simulink model "gm_uz_pmsm_model_6LUT_pd_vnl"  (R2023a)
settings: Solver=FixedStepAuto  StartTime=0.0  StopTime=0.05  RelTol=1e-3
PreLoadFcn:
  | uz_pmsm_model_init_parameter
PostLoadFcn:
  | % Import the data from Excel for a lookup table
  | FluxMapData = readtable('C:\Users\Philipp\ultrazohm\ultrazohm_sw\ip_cores\uz_pmsm_model\FluxMapData_2023-05-26_13-07-57.csv');
  | % Row indices for lookup table
  | d_current_in_d_axis = FluxMapData(8:27,1:end);
  | % Column indices for lookup table
  | q_current_in_d_axis = FluxMapData(29:48,1:end);
  | % Output values for lookup table
  | d_Flux_d_axis = FluxMapData(50:69,1:end);
undefined symbols (not defined in the file or in its folder): d_current_d_Flux, d_current_q_Flux, entkopplung_dynamic, entkopplung_linear, entkopplung_static, Flux_d, Flux_q, friction_coefficient, inertia, k_i_d, k_p_d, k_p_q, Ki_Bo_d, Ki_Bo_q, Kp_Bo_d, Kp_Bo_q, L_d, L_q, Ldd, Ldq, Lqd, Lqq, parameter_nachfuerung, polepair, praediktion_entkopplung_nonlinear, psi_pm, q_current_d_Flux, q_current_q_Flux, R_1, simulate_mechanical, simulate_nonlinear_modell, simulate_open_loop, static_friction_torque, tau_sum, ts, ts_regler
libraries: hdlmdlgenlib x5, slpidlib x4, simulink x2
(part 1 of 2)
settings Model: Creator=ts  LastModifiedBy=Philipp
settings SolverCC: AlgebraicLoopSolver=TrustRegion  AutoInsertRateTranBlk=on
settings DataIOCC: LimitDataPoints=on  SaveOutput=off  SaveTime=off
settings OptimizationCC: BlockReduction=off  ConditionallyExecuteInputs=off  DefaultParameterBehavior=Inlined  LifeSpan=inf
settings DebuggingCC: AlgebraicLoopMsg=error  InheritedTsInSrcMsg=none  SingleTaskRateTransMsg=error  UnconnectedInputMsg=warning  UnconnectedOutputMsg=warning  UnconnectedLineMsg=warning  AllowSymbolicDim=off  StrictBusMsg=ErrorOnBusTreatedAsVector  SFUnexpectedBacktrackingDiag=warning  SFNoUnconditionalDefaultTransitionDiag=warning  SFExecutionAtInitializationDiag=none  ArithmeticOperatorsInVariantConditions=warning
settings HardwareCC: ProdBitPerPointer=32  ProdBitPerSizeT=32  ProdBitPerPtrDiffT=32  ProdLargestAtomicFloat=None  ProdIntDivRoundTo=Undefined  ProdEndianess=Unspecified  ProdWordSize=32  ProdHWDeviceType=ASIC/FPGA->ASIC/FPGA  ProdEqTarget=off
settings ModelReferenceCC: EnableRefExpFcnMdlSchedulingChecks=on
settings SFSimCC: SimUseLocalCustomCode=off  CustomCodeUndefinedFunction=UseInterfaceOnly
settings RTWCC: RTWUseLocalCustomCode=off  DLArmComputeVersion=19.05
settings CodeAppCC: StateflowObjectComments=on
settings GRTTargetCC: TargetLangStandard=C89/C90 (ANSI)
settings ConfigComp: CovScope=ReferencedModels  CovMetricSettings=dw  CovSaveCumulativeToWorkspaceVar=on  CovSaveSingleToWorkspaceVar=on  CovExternalEMLEnable=off  CovSFcnEnable=off

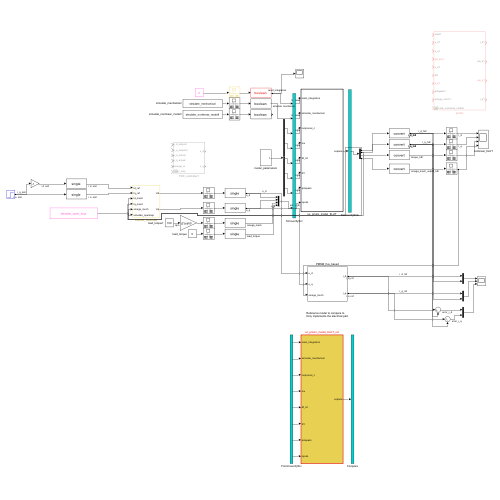
[thumbnail: Simulink's stored preview of the top-level diagram]
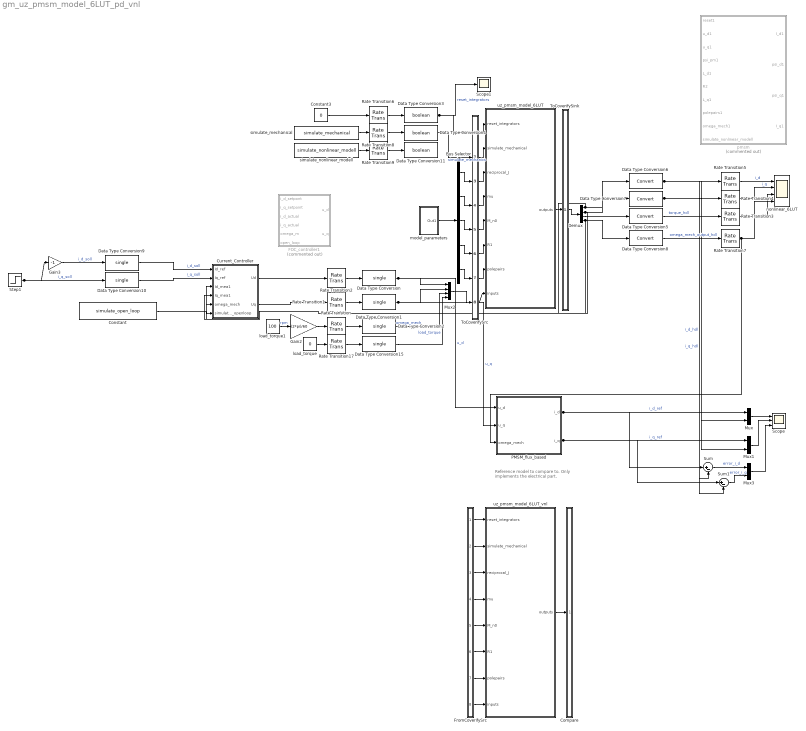
== system gm_uz_pmsm_model_6LUT_pd_vnl ==
  note: Reference model to compare to.
      | Only implements the electrical part.
  Bus Selector : BusSelector  OutputSignals=1_J,mu,M_R0,R_1,polepair
  Compare : Subsystem
      mask Display: disp('')
  Constant : Constant  Value=simulate_open_loop
  Constant3 : Constant  Value=0
  Current_Controller : Subsystem
  Data Type Conversion{,1..2,9..10,15} (6 alike) : DataTypeConversion  OutDataTypeStr=single  SaturateOnIntegerOverflow=off  RndMeth=Floor
  Data Type Conversion11 : DataTypeConversion  OutDataTypeStr=boolean  SaturateOnIntegerOverflow=off  RndMeth=Floor
  Data Type Conversion3 : DataTypeConversion  OutDataTypeStr=boolean  SaturateOnIntegerOverflow=off  RndMeth=Floor
  Data Type Conversion4 : DataTypeConversion  OutDataTypeStr=boolean  SaturateOnIntegerOverflow=off  RndMeth=Floor
  Data Type Conversion{5..8} (4 alike) : DataTypeConversion  SaturateOnIntegerOverflow=off  RndMeth=Floor
  Demux : Demux
  FOC_controller1 : Subsystem  Commented=on
  FromCoverifySrc : Subsystem
      mask Display: disp('')
  Gain2 : Gain  Gain=(2*pi)/60
  Gain3 : Gain  Gain=-1
  Mux : Mux  Inputs=2
  Mux1 : Mux  Inputs=2
  Mux2 : Mux
  Mux3 : Mux  Inputs=2
  PMSM_flux_based : Subsystem
  Rate Transition{,1..2,6,8..9,17} (7 alike) : RateTransition  OutPortSampleTime=ts
  Rate Transition{3..5,7} (4 alike) : RateTransition
  Scope : Scope  NumInputPorts=3
  Scope1 : Scope
  Step1 : Step  Time=0.025
  Sum : Sum  Inputs=|+-
  Sum1 : Sum  Inputs=|+-
  ToCoverifySink : Subsystem
      mask Display: disp('')
  ToCoverifySrc : Subsystem
      mask Display: disp('')
  load_torque : Constant  Value=0
  load_torque1 : Constant  Value=100
  model_parameters : Subsystem
  nonlinear_6LUT : Scope  NumInputPorts=4
  pmsm : Subsystem  Commented=on
  simulate_mechanical : Constant  Value=simulate_mechanical
  simulate_nonlinear_modell : Constant  Value=simulate_nonlinear_modell
  uz_pmsm_model_6LUT : Subsystem  TreatAsAtomicUnit=on
  uz_pmsm_model_6LUT_vnl : Subsystem  TreatAsAtomicUnit=on
  wires:
  Rate Transition/1 -> Data Type Conversion2/1
  Rate Transition1/1 -> Data Type Conversion1/1
  Rate Transition2/1 -> Data Type Conversion/1
  Data Type Conversion6/1 -> Mux/2, Sum/2, Rate Transition5/1  "i_d_hdl"
  Data Type Conversion7/1 -> Rate Transition4/1, Mux1/2, Sum1/2  "i_q_hdl"
  Data Type Conversion5/1 -> Rate Transition3/1  "torque_hdl"
  Rate Transition4/1 -> nonlinear_6LUT/2  "i_q"
  Rate Transition5/1 -> nonlinear_6LUT/1  "i_d"
  Rate Transition3/1 -> nonlinear_6LUT/3
  Rate Transition6/1 -> Data Type Conversion3/1
  Constant3/1 -> Rate Transition6/1
  Rate Transition8/1 -> Data Type Conversion4/1
  simulate_mechanical/1 -> Rate Transition8/1
  Data Type Conversion3/1 -> Scope1/1, ToCoverifySrc/1(in1)  "reset_integrators"
  load_torque/1 -> Rate Transition17/1
  Rate Transition17/1 -> Data Type Conversion15/1
  Mux/1 -> Scope/1
  Mux1/1 -> Scope/2
  PMSM_flux_based/2(i_q) -> Mux1/1, Sum1/1  "i_q_ref"
  PMSM_flux_based/1(i_d) -> Mux/1, Sum/1  "i_d_ref"
  Data Type Conversion8/1 -> Rate Transition7/1  "omega_mech_output_hdl"
  Rate Transition7/1 -> PMSM_flux_based/3(omega_mech), nonlinear_6LUT/4
  model_parameters/1(Out1) -> Bus Selector/1
  Sum/1 -> Mux3/1  "error_i_d"
  Sum1/1 -> Mux3/2  "error_i_q"
  Mux3/1 -> Scope/3
  Step1/1 -> Gain3/1, Data Type Conversion10/1  "i_q_soll"
  Demux/3 -> Data Type Conversion5/1
  Gain3/1 -> Data Type Conversion9/1  "i_d_soll"
  Demux/1 -> Current_Controller/3(Id_mea1), Data Type Conversion6/1
  Demux/4 -> Current_Controller/5(omega_mech), Data Type Conversion8/1
  Demux/2 -> Current_Controller/4(Iq_mea1), Data Type Conversion7/1
  Data Type Conversion/1 -> PMSM_flux_based/1(u_d), Mux2/1  "u_d"
  Data Type Conversion1/1 -> PMSM_flux_based/2(u_q), Mux2/2  "u_q"
  Data Type Conversion15/1 -> Mux2/4  "load_torque"
  Data Type Conversion2/1 -> Mux2/3  "omega_mech"
  Data Type Conversion9/1 -> Current_Controller/1(Id_ref)  "i_d_soll"
  Data Type Conversion10/1 -> Current_Controller/2(Iq_ref)  "i_q_soll"
  Current_Controller/1(Ud) -> Rate Transition2/1
  Current_Controller/2(Uq) -> Rate Transition1/1
  Gain2/1 -> Rate Transition/1
  Constant/1 -> Current_Controller/6(simulate_openloop)
  load_torque1/1 -> Gain2/1  "rpm"
  simulate_nonlinear_modell/1 -> Rate Transition9/1
  Rate Transition9/1 -> Data Type Conversion11/1
  ToCoverifySrc/1(out1) -> uz_pmsm_model_6LUT/1(reset_integrators)
  ToCoverifySrc/2(out2) -> uz_pmsm_model_6LUT/2(simulate_mechanical)
  ToCoverifySrc/3(out3) -> uz_pmsm_model_6LUT/3(reciprocal_J)
  ToCoverifySrc/4(out4) -> uz_pmsm_model_6LUT/4(mu)
  ToCoverifySrc/5(out5) -> uz_pmsm_model_6LUT/5(M_n0)
  ToCoverifySrc/6(out6) -> uz_pmsm_model_6LUT/6(R1)
  ToCoverifySrc/7(out7) -> uz_pmsm_model_6LUT/7(polepairs)
  ToCoverifySrc/8(out8) -> uz_pmsm_model_6LUT/8(inputs)
  uz_pmsm_model_6LUT/1(outputs) -> ToCoverifySink/1(in1)
  Data Type Conversion4/1 -> ToCoverifySrc/2(in2)  "simulate_mechanics"
  Bus Selector/1 -> ToCoverifySrc/3(in3)
  Bus Selector/2 -> ToCoverifySrc/4(in4)
  Bus Selector/3 -> ToCoverifySrc/5(in5)
  Bus Selector/4 -> ToCoverifySrc/6(in6)
  Bus Selector/5 -> ToCoverifySrc/7(in7)
  Mux2/1 -> ToCoverifySrc/8(in8)
  ToCoverifySink/1(out1) -> Demux/1
  FromCoverifySrc/1(out1) -> uz_pmsm_model_6LUT_vnl/1(reset_integrators)
  FromCoverifySrc/2(out2) -> uz_pmsm_model_6LUT_vnl/2(simulate_mechanical)
  FromCoverifySrc/3(out3) -> uz_pmsm_model_6LUT_vnl/3(reciprocal_J)
  FromCoverifySrc/4(out4) -> uz_pmsm_model_6LUT_vnl/4(mu)
  FromCoverifySrc/5(out5) -> uz_pmsm_model_6LUT_vnl/5(M_n0)
  FromCoverifySrc/6(out6) -> uz_pmsm_model_6LUT_vnl/6(R1)
  FromCoverifySrc/7(out7) -> uz_pmsm_model_6LUT_vnl/7(polepairs)
  FromCoverifySrc/8(out8) -> uz_pmsm_model_6LUT_vnl/8(inputs)
  uz_pmsm_model_6LUT_vnl/1(outputs) -> Compare/1(in1)

== system gm_uz_pmsm_model_6LUT_pd_vnl/Compare ==
  in1 : Inport
  Assert_outputs : Subsystem  mask{ToleranceValue=1e-07}
      settings: LibrarySourceBlock=hdlmdlgenlib/AssertRelEqIDC
  CleanupScopes : Subsystem
      settings: OpenFcn=|
      | blkName = gcb; %self block
      | idx = regexp(blkName, '/CleanupScopes$', 'once');
      | blkParent = blkName(1:idx-1);
      | blks=find_system(blkParent, 'LookUnderMasks', 'all','blocktype', 'Scope');
      | for itr = 1:length(blks)
      | 	 hScopeCfg = get_param(blks{itr},'ScopeConfiguration');
      | 	 hScopeCfg.Visible = ~ hScopeCfg.Visible;
      | end
      | drawnow;
      mask Display: fprintf(message('hdlcoder:cosim:vnl_dblclick').getString());
  Enable : Subsystem
      settings: OpenFcn=|
      | blkName = gcb;
      | idx = regexp(blkName, '/Enable$', 'once');
      | blkParent = blkName(1:idx-1);
      | blks=find_system(blkParent, 'LookUnderMasks', 'all','blocktype', 'Assertion');
      | e = get_param(blks{1}, 'Enabled');
      | if strcmp(e, 'on'), f= 'off';, else, f = 'on';, end
      | for ii=1:length(blks), set_param(blks{ii}, 'Enabled', f);, end
      | set_param(gcb, 'MaskDisplay',['fprintf(message(''hdlcoder:cosim:vnl_dblclick_assertions'',','''',upper(e),'''',').getString())']);
      mask Display: fprintf(message('hdlcoder:cosim:vnl_dblclick_assertions','OFF').getString());
  pathdelay1 : Delay  DelayLength=1
  wires:
  in1/1 -> pathdelay1/1
  pathdelay1/1 -> Assert_outputs/1(cosim)
  [out1] -> Assert_outputs/2(dut)

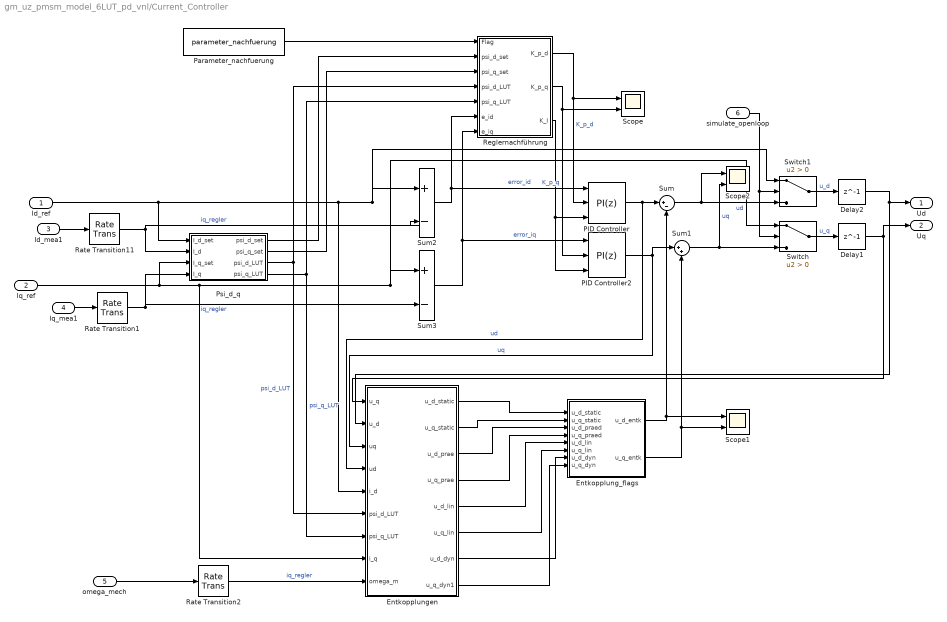
== system gm_uz_pmsm_model_6LUT_pd_vnl/Current_Controller ==
  Id_ref : Inport
  Iq_ref : Inport  Port=2
  Id_mea1 : Inport  Port=3
  Iq_mea1 : Inport  Port=4
  omega_mech : Inport  Port=5
  simulate_openloop : Inport  Port=6
  Delay1 : Delay  DelayLength=1
  Delay2 : Delay  DelayLength=1
  Entkopplung_flags : Subsystem
  Entkopplungen : Subsystem
  PID Controller : slpidlib/PID Controller  Controller=PI  Form=Parallel  TimeDomain=Discrete-time  UseExternalTs=off  SampleTime=-1  IntegratorMethod=Forward Euler  FilterMethod=Forward Euler  ControllerParametersSource=external  P=Kp_Bo_d  I=Ki_Bo_d  UseKiTs=off  D=0  N=100  UseFilter=on  TunerSelectOption=Transfer Function Based (PID Tuner App)  InitialConditionSource=internal  InitialConditionForIntegrator=0  InitialConditionForFilter=0  DifferentiatorICPrevScaledInput=0  ExternalReset=none  TrackingMode=off  Kt=1  LimitOutput=off  SatLimitsSource=internal  UpperSaturationLimit=48  LowerSaturationLimit=-48  LinearizeAsGain=off  AntiWindupMode=clamping  Kb=1  LimitIntegrator=off  UpperIntegratorSaturationLimit=48  LowerIntegratorSaturationLimit=-48  POutMin=[]  POutMax=[]  IOutMin=[]  IOutMax=[]  DOutMin=[]  DOutMax=[]  NOutMin=[]  NOutMax=[]  SumOutMin=[]  SumOutMax=[]  SaturationOutMin=[]  SaturationOutMax=[]  PParamMin=[]  PParamMax=[]  IParamMin=[]  IParamMax=[]  DParamMin=[]  DParamMax=[]  NParamMin=[]  NParamMax=[]  KbParamMin=[]  KbParamMax=[]  KtParamMin=[]  KtParamMax=[]  KbOutMin=[]  KbOutMax=[]  KtOutMin=[]  KtOutMax=[]  IntegratorOutMin=[]  IntegratorOutMax=[]  FilterOutMin=[]  FilterOutMax=[]  SumI1OutMin=[]  SumI1OutMax=[]  SumI2OutMin=[]  SumI2OutMax=[]  SumI3OutMin=[]  SumI3OutMax=[]  SumI4OutMin=[]  SumI4OutMax=[]  SumDOutMin=[]  SumDOutMax=[]  DifferentiatorOutMin=[]  DifferentiatorOutMax=[]  FilterDiffOutCoefMin=[]  FilterDiffOutCoefMax=[]  ReciprocalOutMin=[]  ReciprocalOutMax=[]  SumDenOutMin=[]  SumDenOutMax=[]  SumNumOutMin=[]  SumNumOutMax=[]  DivideOutMin=[]  DivideOutMax=[]  UdiffTsProdOutMin=[]  UdiffTsProdOutMax=[]  NTsProdOutMin=[]  NTsProdOutMax=[]  UintegralTsProdOutMin=[]  UintegralTsProdOutMax=[]  UngainTsProdOutMin=[]  UngainTsProdOutMax=[]  ClampingZeroOutDataTypeStr=Inherit: Inherit via back propagation  ClampingZeroOutMin=[]  ClampingZeroOutMax=[]  FilterDenConstantOutDataTypeStr=Inherit: Inherit via back propagation  FilterDenConstantOutMin=[]  FilterDenConstantOutMax=[]  PCopyOutDataTypeStr=Inherit: Inherit via back propagation  PCopyOutMin=[]  PCopyOutMax=[]  NCopyOutDataTypeStr=Inherit: Inherit via back propagation  NCopyOutMin=[]  NCopyOutMax=[]  IntegratorContinuousStateAttributes=''  IntegratorStateMustResolveToSignalObject=off  IntegratorRTWStateStorageClass=Auto  FilterContinuousStateAttributes=''  FilterStateMustResolveToSignalObject=off  FilterRTWStateStorageClass=Auto  ParallelPVariant=ExternalParameters  IdealPVariant=Disabled  IVariant=ExternalParameters  DVariant=Disabled  IntegratorVariant=Discrete  SatVariant=Disabled  AWVariant=Passthrough  PCopyVariant=Disabled  TRVariant=Disabled  FdbkBlocksVariant=Forward  IdealPFdbkVariant=Disabled  SatFdbkVariant=Disabled  DerivativeFilterVariant=Disabled  NVariant=Disabled  NCopyVariant=Disabled_SignalSpec  FilterICVariant=Disabled  IntegratorICVariant=InternalICs  ExternalResetVariant=Disabled  TRSumVariant=Passthrough  SumFdbkVariant=Disabled  SumVariant=Sum_PI  TsampFilterVariant=InternalTs  TsampNgainVariant=Passthrough  TsampIntegralVariant=Disabled_SignalSpec  ExternalSaturationOutDataTypeStr=Inherit: Same as second input
  PID Controller2 : slpidlib/PID Controller  Controller=PI  Form=Parallel  TimeDomain=Discrete-time  UseExternalTs=off  SampleTime=-1  IntegratorMethod=Forward Euler  FilterMethod=Forward Euler  ControllerParametersSource=external  P=Kp_Bo_q  I=Ki_Bo_q  UseKiTs=off  D=0  N=100  UseFilter=on  TunerSelectOption=Transfer Function Based (PID Tuner App)  InitialConditionSource=internal  InitialConditionForIntegrator=0  InitialConditionForFilter=0  DifferentiatorICPrevScaledInput=0  ExternalReset=none  TrackingMode=off  Kt=1  LimitOutput=off  SatLimitsSource=internal  UpperSaturationLimit=48  LowerSaturationLimit=-48  LinearizeAsGain=off  AntiWindupMode=clamping  Kb=1  LimitIntegrator=off  UpperIntegratorSaturationLimit=48  LowerIntegratorSaturationLimit=-48  POutMin=[]  POutMax=[]  IOutMin=[]  IOutMax=[]  DOutMin=[]  DOutMax=[]  NOutMin=[]  NOutMax=[]  SumOutMin=[]  SumOutMax=[]  SaturationOutMin=[]  SaturationOutMax=[]  PParamMin=[]  PParamMax=[]  IParamMin=[]  IParamMax=[]  DParamMin=[]  DParamMax=[]  NParamMin=[]  NParamMax=[]  KbParamMin=[]  KbParamMax=[]  KtParamMin=[]  KtParamMax=[]  KbOutMin=[]  KbOutMax=[]  KtOutMin=[]  KtOutMax=[]  IntegratorOutMin=[]  IntegratorOutMax=[]  FilterOutMin=[]  FilterOutMax=[]  SumI1OutMin=[]  SumI1OutMax=[]  SumI2OutMin=[]  SumI2OutMax=[]  SumI3OutMin=[]  SumI3OutMax=[]  SumI4OutMin=[]  SumI4OutMax=[]  SumDOutMin=[]  SumDOutMax=[]  DifferentiatorOutMin=[]  DifferentiatorOutMax=[]  FilterDiffOutCoefMin=[]  FilterDiffOutCoefMax=[]  ReciprocalOutMin=[]  ReciprocalOutMax=[]  SumDenOutMin=[]  SumDenOutMax=[]  SumNumOutMin=[]  SumNumOutMax=[]  DivideOutMin=[]  DivideOutMax=[]  UdiffTsProdOutMin=[]  UdiffTsProdOutMax=[]  NTsProdOutMin=[]  NTsProdOutMax=[]  UintegralTsProdOutMin=[]  UintegralTsProdOutMax=[]  UngainTsProdOutMin=[]  UngainTsProdOutMax=[]  ClampingZeroOutDataTypeStr=Inherit: Inherit via back propagation  ClampingZeroOutMin=[]  ClampingZeroOutMax=[]  FilterDenConstantOutDataTypeStr=Inherit: Inherit via back propagation  FilterDenConstantOutMin=[]  FilterDenConstantOutMax=[]  PCopyOutDataTypeStr=Inherit: Inherit via back propagation  PCopyOutMin=[]  PCopyOutMax=[]  NCopyOutDataTypeStr=Inherit: Inherit via back propagation  NCopyOutMin=[]  NCopyOutMax=[]  IntegratorContinuousStateAttributes=''  IntegratorStateMustResolveToSignalObject=off  IntegratorRTWStateStorageClass=Auto  FilterContinuousStateAttributes=''  FilterStateMustResolveToSignalObject=off  FilterRTWStateStorageClass=Auto  ParallelPVariant=ExternalParameters  IdealPVariant=Disabled  IVariant=ExternalParameters  DVariant=Disabled  IntegratorVariant=Discrete  SatVariant=Disabled  AWVariant=Passthrough  PCopyVariant=Disabled  TRVariant=Disabled  FdbkBlocksVariant=Forward  IdealPFdbkVariant=Disabled  SatFdbkVariant=Disabled  DerivativeFilterVariant=Disabled  NVariant=Disabled  NCopyVariant=Disabled_SignalSpec  FilterICVariant=Disabled  IntegratorICVariant=InternalICs  ExternalResetVariant=Disabled  TRSumVariant=Passthrough  SumFdbkVariant=Disabled  SumVariant=Sum_PI  TsampFilterVariant=InternalTs  TsampNgainVariant=Passthrough  TsampIntegralVariant=Disabled_SignalSpec  ExternalSaturationOutDataTypeStr=Inherit: Same as second input
  Parameter_nachfuerung : Constant  Value=parameter_nachfuerung
  Psi_d_q : Subsystem
  Rate Transition1 : RateTransition  OutPortSampleTime=ts_regler
  Rate Transition11 : RateTransition  OutPortSampleTime=ts_regler
  Rate Transition2 : RateTransition  OutPortSampleTime=ts_regler
  Reglernachführung : Subsystem
  Scope : Scope  NumInputPorts=2
  Scope1 : Scope  NumInputPorts=2
  Scope2 : Scope  NumInputPorts=2
  Sum : Sum  Inputs=|+-
  Sum1 : Sum  Inputs=|++
  Sum2 : Sum  Inputs=|+-
  Sum3 : Sum  Inputs=|+-
  Switch : Switch  Criteria=u2 > Threshold  SaturateOnIntegerOverflow=off  InputSameDT=off
  Switch1 : Switch  Criteria=u2 > Threshold  SaturateOnIntegerOverflow=off  InputSameDT=off
  Ud : Outport
  Uq : Outport  Port=2
  wires:
  Sum3/1 -> Reglernachführung/7(e_iq), PID Controller2/1  "error_iq"
  Sum2/1 -> PID Controller/1, Reglernachführung/6(e_id)  "error_id"
  Sum/1 -> Scope2/1, Switch1/3  "ud"
  PID Controller/1 -> Entkopplungen/4(ud), Sum/1  "ud"
  PID Controller2/1 -> Sum1/1, Entkopplungen/3(uq)  "uq"
  Sum1/1 -> Scope2/2, Switch/3  "uq"
  Iq_ref/1 -> Entkopplungen/8(i_q), Sum3/1, Switch/1, Psi_d_q/3(I_q_set)
  Id_ref/1 -> Psi_d_q/1(I_d_set), Entkopplungen/5(i_d), Sum2/1, Switch1/1
  Switch/1 -> Delay1/1  "u_q"
  Switch1/1 -> Delay2/1  "u_d"
  simulate_openloop/1 -> Switch/2, Switch1/2
  Reglernachführung/1(K_p_d) -> PID Controller/2, Scope/1  "K_p_d"
  Reglernachführung/2(K_p_q) -> PID Controller2/2, Scope/2  "K_p_q"
  Reglernachführung/3(K_I) -> PID Controller2/3, PID Controller/3
  Id_mea1/1 -> Rate Transition11/1
  Iq_mea1/1 -> Rate Transition1/1
  Psi_d_q/3(psi_d_LUT) -> Reglernachführung/4(psi_d_LUT), Entkopplungen/6(psi_d_LUT)  "psi_d_LUT"
  Psi_d_q/4(psi_q_LUT) -> Reglernachführung/5(psi_q_LUT), Entkopplungen/7(psi_q_LUT)  "psi_q_LUT"
  Parameter_nachfuerung/1 -> Reglernachführung/1(Flag)
  Psi_d_q/1(psi_d_set) -> Reglernachführung/2(psi_d_set)
  Psi_d_q/2(psi_q_set) -> Reglernachführung/3(psi_q_set)
  omega_mech/1 -> Rate Transition2/1
  Entkopplungen/1(u_d_static) -> Entkopplung_flags/1(u_d_static)
  Entkopplungen/2(u_q_static) -> Entkopplung_flags/2(u_q_static)
  Entkopplungen/3(u_d_prae) -> Entkopplung_flags/3(u_d_praed)
  Entkopplungen/4(u_q_prae) -> Entkopplung_flags/4(u_q_praed)
  Entkopplungen/5(u_d_lin) -> Entkopplung_flags/5(u_d_lin)
  Entkopplungen/6(u_q_lin) -> Entkopplung_flags/6(u_q_lin)
  Entkopplung_flags/1(u_d_entk) -> Scope1/1, Sum/2
  Entkopplung_flags/2(u_q_entk) -> Scope1/2, Sum1/2
  Rate Transition11/1 -> Sum2/2, Psi_d_q/2(I_d)  "iq_regler"
  Rate Transition1/1 -> Sum3/2, Psi_d_q/4(I_q)  "iq_regler"
  Rate Transition2/1 -> Entkopplungen/9(omega_m)  "iq_regler"
  Delay2/1 -> Ud/1, Entkopplungen/2(u_d)
  Delay1/1 -> Uq/1, Entkopplungen/1(u_q)
  Entkopplungen/7(u_d_dyn) -> Entkopplung_flags/7(u_d_dyn)
  Entkopplungen/8(u_q_dyn1) -> Entkopplung_flags/8(u_q_dyn)

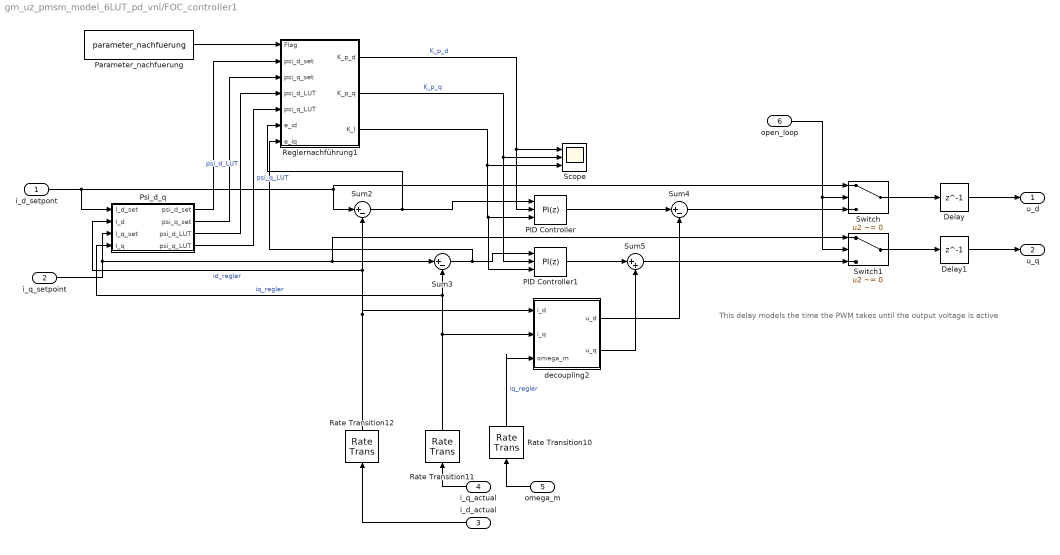
== system gm_uz_pmsm_model_6LUT_pd_vnl/FOC_controller1 ==
  note: This delay models the time the PWM takes until the output voltage is active
  i_d_setpont : Inport
  i_q_setpoint : Inport  Port=2
  i_d_actual : Inport  Port=3
  i_q_actual : Inport  Port=4
  omega_m : Inport  Port=5
  open_loop : Inport  Port=6
  Delay : Delay  DelayLength=1
  Delay1 : Delay  DelayLength=1
  PID Controller : slpidlib/PID Controller  Controller=PI  Form=Parallel  TimeDomain=Discrete-time  UseExternalTs=off  SampleTime=-1  IntegratorMethod=Forward Euler  FilterMethod=Forward Euler  ControllerParametersSource=external  P=k_p_d  I=k_i_d  UseKiTs=off  D=0  N=100  UseFilter=on  TunerSelectOption=Transfer Function Based (PID Tuner App)  InitialConditionSource=internal  InitialConditionForIntegrator=0  InitialConditionForFilter=0  DifferentiatorICPrevScaledInput=0  ExternalReset=none  TrackingMode=off  Kt=1  LimitOutput=off  SatLimitsSource=internal  UpperSaturationLimit=48  LowerSaturationLimit=-48  LinearizeAsGain=on  AntiWindupMode=clamping  Kb=1  LimitIntegrator=off  UpperIntegratorSaturationLimit=inf  LowerIntegratorSaturationLimit=-inf  POutMin=[]  POutMax=[]  IOutMin=[]  IOutMax=[]  DOutMin=[]  DOutMax=[]  NOutMin=[]  NOutMax=[]  SumOutMin=[]  SumOutMax=[]  SaturationOutMin=[]  SaturationOutMax=[]  PParamMin=[]  PParamMax=[]  IParamMin=[]  IParamMax=[]  DParamMin=[]  DParamMax=[]  NParamMin=[]  NParamMax=[]  KbParamMin=[]  KbParamMax=[]  KtParamMin=[]  KtParamMax=[]  KbOutMin=[]  KbOutMax=[]  KtOutMin=[]  KtOutMax=[]  IntegratorOutMin=[]  IntegratorOutMax=[]  FilterOutMin=[]  FilterOutMax=[]  SumI1OutMin=[]  SumI1OutMax=[]  SumI2OutMin=[]  SumI2OutMax=[]  SumI3OutMin=[]  SumI3OutMax=[]  SumI4OutMin=[]  SumI4OutMax=[]  SumDOutMin=[]  SumDOutMax=[]  DifferentiatorOutMin=[]  DifferentiatorOutMax=[]  FilterDiffOutCoefMin=[]  FilterDiffOutCoefMax=[]  ReciprocalOutMin=[]  ReciprocalOutMax=[]  SumDenOutMin=[]  SumDenOutMax=[]  SumNumOutMin=[]  SumNumOutMax=[]  DivideOutMin=[]  DivideOutMax=[]  UdiffTsProdOutMin=[]  UdiffTsProdOutMax=[]  NTsProdOutMin=[]  NTsProdOutMax=[]  UintegralTsProdOutMin=[]  UintegralTsProdOutMax=[]  UngainTsProdOutMin=[]  UngainTsProdOutMax=[]  ClampingZeroOutDataTypeStr=Inherit: Inherit via back propagation  ClampingZeroOutMin=[]  ClampingZeroOutMax=[]  FilterDenConstantOutDataTypeStr=Inherit: Inherit via back propagation  FilterDenConstantOutMin=[]  FilterDenConstantOutMax=[]  PCopyOutDataTypeStr=Inherit: Inherit via back propagation  PCopyOutMin=[]  PCopyOutMax=[]  NCopyOutDataTypeStr=Inherit: Inherit via back propagation  NCopyOutMin=[]  NCopyOutMax=[]  IntegratorContinuousStateAttributes=''  IntegratorStateMustResolveToSignalObject=off  IntegratorRTWStateStorageClass=Auto  FilterContinuousStateAttributes=''  FilterStateMustResolveToSignalObject=off  FilterRTWStateStorageClass=Auto  ParallelPVariant=ExternalParameters  IdealPVariant=Disabled  IVariant=ExternalParameters  DVariant=Disabled  IntegratorVariant=Discrete  SatVariant=Disabled  AWVariant=Passthrough  PCopyVariant=Disabled  TRVariant=Disabled  FdbkBlocksVariant=Forward  IdealPFdbkVariant=Disabled  SatFdbkVariant=Disabled  DerivativeFilterVariant=Disabled  NVariant=Disabled  NCopyVariant=Disabled_SignalSpec  FilterICVariant=Disabled  IntegratorICVariant=InternalICs  ExternalResetVariant=Disabled  TRSumVariant=Passthrough  SumFdbkVariant=Disabled  SumVariant=Sum_PI  TsampFilterVariant=InternalTs  TsampNgainVariant=Passthrough  TsampIntegralVariant=Disabled_SignalSpec  ExternalSaturationOutDataTypeStr=Inherit: Same as second input
  PID Controller1 : slpidlib/PID Controller  Controller=PI  Form=Parallel  TimeDomain=Discrete-time  UseExternalTs=off  SampleTime=-1  IntegratorMethod=Forward Euler  FilterMethod=Forward Euler  ControllerParametersSource=external  P=k_p_q  I=k_i_d  UseKiTs=off  D=0  N=100  UseFilter=on  TunerSelectOption=Transfer Function Based (PID Tuner App)  InitialConditionSource=internal  InitialConditionForIntegrator=0  InitialConditionForFilter=0  DifferentiatorICPrevScaledInput=0  ExternalReset=none  TrackingMode=off  Kt=1  LimitOutput=off  SatLimitsSource=internal  UpperSaturationLimit=48  LowerSaturationLimit=-48  LinearizeAsGain=on  AntiWindupMode=clamping  Kb=1  LimitIntegrator=off  UpperIntegratorSaturationLimit=inf  LowerIntegratorSaturationLimit=-inf  POutMin=[]  POutMax=[]  IOutMin=[]  IOutMax=[]  DOutMin=[]  DOutMax=[]  NOutMin=[]  NOutMax=[]  SumOutMin=[]  SumOutMax=[]  SaturationOutMin=[]  SaturationOutMax=[]  PParamMin=[]  PParamMax=[]  IParamMin=[]  IParamMax=[]  DParamMin=[]  DParamMax=[]  NParamMin=[]  NParamMax=[]  KbParamMin=[]  KbParamMax=[]  KtParamMin=[]  KtParamMax=[]  KbOutMin=[]  KbOutMax=[]  KtOutMin=[]  KtOutMax=[]  IntegratorOutMin=[]  IntegratorOutMax=[]  FilterOutMin=[]  FilterOutMax=[]  SumI1OutMin=[]  SumI1OutMax=[]  SumI2OutMin=[]  SumI2OutMax=[]  SumI3OutMin=[]  SumI3OutMax=[]  SumI4OutMin=[]  SumI4OutMax=[]  SumDOutMin=[]  SumDOutMax=[]  DifferentiatorOutMin=[]  DifferentiatorOutMax=[]  FilterDiffOutCoefMin=[]  FilterDiffOutCoefMax=[]  ReciprocalOutMin=[]  ReciprocalOutMax=[]  SumDenOutMin=[]  SumDenOutMax=[]  SumNumOutMin=[]  SumNumOutMax=[]  DivideOutMin=[]  DivideOutMax=[]  UdiffTsProdOutMin=[]  UdiffTsProdOutMax=[]  NTsProdOutMin=[]  NTsProdOutMax=[]  UintegralTsProdOutMin=[]  UintegralTsProdOutMax=[]  UngainTsProdOutMin=[]  UngainTsProdOutMax=[]  ClampingZeroOutDataTypeStr=Inherit: Inherit via back propagation  ClampingZeroOutMin=[]  ClampingZeroOutMax=[]  FilterDenConstantOutDataTypeStr=Inherit: Inherit via back propagation  FilterDenConstantOutMin=[]  FilterDenConstantOutMax=[]  PCopyOutDataTypeStr=Inherit: Inherit via back propagation  PCopyOutMin=[]  PCopyOutMax=[]  NCopyOutDataTypeStr=Inherit: Inherit via back propagation  NCopyOutMin=[]  NCopyOutMax=[]  IntegratorContinuousStateAttributes=''  IntegratorStateMustResolveToSignalObject=off  IntegratorRTWStateStorageClass=Auto  FilterContinuousStateAttributes=''  FilterStateMustResolveToSignalObject=off  FilterRTWStateStorageClass=Auto  ParallelPVariant=ExternalParameters  IdealPVariant=Disabled  IVariant=ExternalParameters  DVariant=Disabled  IntegratorVariant=Discrete  SatVariant=Disabled  AWVariant=Passthrough  PCopyVariant=Disabled  TRVariant=Disabled  FdbkBlocksVariant=Forward  IdealPFdbkVariant=Disabled  SatFdbkVariant=Disabled  DerivativeFilterVariant=Disabled  NVariant=Disabled  NCopyVariant=Disabled_SignalSpec  FilterICVariant=Disabled  IntegratorICVariant=InternalICs  ExternalResetVariant=Disabled  TRSumVariant=Passthrough  SumFdbkVariant=Disabled  SumVariant=Sum_PI  TsampFilterVariant=InternalTs  TsampNgainVariant=Passthrough  TsampIntegralVariant=Disabled_SignalSpec  ExternalSaturationOutDataTypeStr=Inherit: Same as second input
  Parameter_nachfuerung : Constant  Value=parameter_nachfuerung
  Psi_d_q : Subsystem
  Rate Transition10 : RateTransition  OutPortSampleTime=ts_regler
  Rate Transition11 : RateTransition  OutPortSampleTime=ts_regler
  Rate Transition12 : RateTransition  OutPortSampleTime=ts_regler
  Reglernachführung1 : Subsystem
  Scope : Scope  NumInputPorts=3
  Sum2 : Sum  Inputs=|+-
  Sum3 : Sum  Inputs=|+-
  Sum4 : Sum  Inputs=|+-
  Sum5 : Sum  Inputs=|++
  Switch : Switch  Criteria=u2 ~= 0  SaturateOnIntegerOverflow=off  InputSameDT=off
  Switch1 : Switch  Criteria=u2 ~= 0  SaturateOnIntegerOverflow=off  InputSameDT=off
  decoupling2 : Subsystem
  u_d : Outport
  u_q : Outport  Port=2
  wires:
  PID Controller/1 -> Sum4/1
  PID Controller1/1 -> Sum5/1
  Sum4/1 -> Switch/3
  i_d_actual/1 -> Rate Transition12/1
  i_d_setpont/1 -> Sum2/1, Switch/1, Psi_d_q/1(I_d_set)
  Sum2/1 -> Reglernachführung1/6(e_id), PID Controller/1
  Sum5/1 -> Switch1/3
  omega_m/1 -> Rate Transition10/1
  Sum3/1 -> Reglernachführung1/7(e_iq), PID Controller1/1
  i_q_actual/1 -> Rate Transition11/1
  Rate Transition12/1 -> Psi_d_q/2(I_d), Sum2/2, decoupling2/1(i_d)  "id_regler"
  Rate Transition11/1 -> Sum3/2, Psi_d_q/4(I_q), decoupling2/2(i_q)  "iq_regler"
  i_q_setpoint/1 -> Switch1/1, Sum3/1, Psi_d_q/3(I_q_set)
  open_loop/1 -> Switch1/2, Switch/2
  Rate Transition10/1 -> decoupling2/3(omega_m)  "iq_regler"
  decoupling2/1(u_d) -> Sum4/2
  decoupling2/2(u_q) -> Sum5/2
  Switch/1 -> Delay/1
  Switch1/1 -> Delay1/1
  Delay/1 -> u_d/1
  Delay1/1 -> u_q/1
  Reglernachführung1/1(K_p_d) -> PID Controller/2, Scope/1  "K_p_d"
  Reglernachführung1/2(K_p_q) -> PID Controller1/2, Scope/2  "K_p_q"
  Reglernachführung1/3(K_I) -> PID Controller1/3, PID Controller/3, Scope/3
  Psi_d_q/1(psi_d_set) -> Reglernachführung1/2(psi_d_set)
  Psi_d_q/2(psi_q_set) -> Reglernachführung1/3(psi_q_set)
  Psi_d_q/3(psi_d_LUT) -> Reglernachführung1/4(psi_d_LUT)  "psi_d_LUT"
  Psi_d_q/4(psi_q_LUT) -> Reglernachführung1/5(psi_q_LUT)  "psi_q_LUT"
  Parameter_nachfuerung/1 -> Reglernachführung1/1(Flag)

== system gm_uz_pmsm_model_6LUT_pd_vnl/FromCoverifySrc ==
  out1 : Outport
  out2 : Outport  Port=2
  out3 : Outport  Port=3
  out4 : Outport  Port=4
  out5 : Outport  Port=5
  out6 : Outport  Port=6
  out7 : Outport  Port=7
  out8 : Outport  Port=8
  wires:
  [in1] -> out1/1
  [in2] -> out2/1
  [in3] -> out3/1
  [in4] -> out4/1
  [in5] -> out5/1
  [in6] -> out6/1
  [in7] -> out7/1
  [in8] -> out8/1

== system gm_uz_pmsm_model_6LUT_pd_vnl/PMSM_flux_based ==
  u_d : Inport
  u_q : Inport  Port=2
  omega_mech : Inport  Port=3
  Constant : Constant  Value=psi_pm
  Gain : Gain  Gain=R_1
  Gain1 : Gain  Gain=1/L_d
  Gain2 : Gain  Gain=R_1
  Gain3 : Gain  Gain=1/L_q
  Gain6 : Gain  Gain=polepair
  Integrator : Integrator
  Integrator1 : Integrator
  Product : Product
  Product1 : Product
  Sum : Sum  Inputs=-++
  Sum1 : Sum  Inputs=-+-
  Sum2 : Sum  Inputs=+-
  i_d : Outport
  i_q : Outport  Port=2
  wires:
  u_d/1 -> Sum/2
  u_q/1 -> Sum1/2
  Sum/1 -> Integrator/1
  Gain/1 -> Sum/1
  Integrator/1 -> Product1/2, Sum2/1
  Constant/1 -> Sum2/2
  Sum2/1 -> Gain1/1
  Gain1/1 -> Gain/1, i_d/1
  Gain6/1 -> Product1/1, Product/1
  Product/1 -> Sum/3
  Integrator1/1 -> Gain3/1, Product/2
  Product1/1 -> Sum1/3
  Sum1/1 -> Integrator1/1
  Gain2/1 -> Sum1/1
  Gain3/1 -> i_q/1, Gain2/1
  omega_mech/1 -> Gain6/1

== system gm_uz_pmsm_model_6LUT_pd_vnl/ToCoverifySink ==
  in1 : Inport
  out1 : Outport
  tag scope: out1=global
  wires:
  in1/1 -> out1/1, [out1]

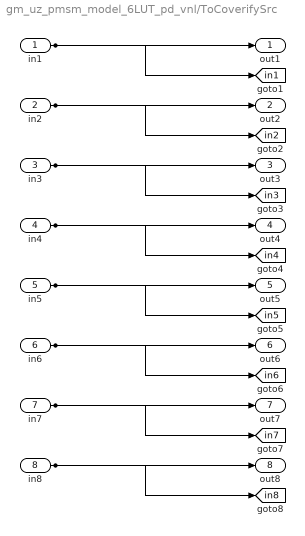
== system gm_uz_pmsm_model_6LUT_pd_vnl/ToCoverifySrc ==
  in1 : Inport
  in2 : Inport  Port=2
  in3 : Inport  Port=3
  in4 : Inport  Port=4
  in5 : Inport  Port=5
  in6 : Inport  Port=6
  in7 : Inport  Port=7
  in8 : Inport  Port=8
  out1 : Outport
  out2 : Outport  Port=2
  out3 : Outport  Port=3
  out4 : Outport  Port=4
  out5 : Outport  Port=5
  out6 : Outport  Port=6
  out7 : Outport  Port=7
  out8 : Outport  Port=8
  tag scope: in1=global, in2=global, in3=global, in4=global, in5=global, in6=global, in7=global, in8=global
  wires:
  in1/1 -> out1/1, [in1]
  in2/1 -> out2/1, [in2]
  in3/1 -> out3/1, [in3]
  in4/1 -> out4/1, [in4]
  in5/1 -> out5/1, [in5]
  in6/1 -> out6/1, [in6]
  in7/1 -> out7/1, [in7]
  in8/1 -> out8/1, [in8]

== system gm_uz_pmsm_model_6LUT_pd_vnl/model_parameters ==
  Bus Creator : BusCreator  Inputs=5
  Constant7 : Constant  Value=R_1
  Constant8 : Constant  Value=polepair
  Data Type Conversion{9..10,12..14} (5 alike) : DataTypeConversion  OutDataTypeStr=single  SaturateOnIntegerOverflow=off  RndMeth=Floor
  J : Constant  Value=1/inertia
  M_R0 : Constant  Value=static_friction_torque
  Rate Transition{10,12..13,15..16} (5 alike) : RateTransition  OutPortSampleTime=ts
  mu : Constant  Value=friction_coefficient
  Out1 : Outport
  wires:
  Data Type Conversion12/1 -> Rate Transition16/1
  Rate Transition10/1 -> Bus Creator/3  "M_R0"
  Data Type Conversion14/1 -> Rate Transition10/1
  Rate Transition12/1 -> Bus Creator/4  "R_1"
  Rate Transition16/1 -> Bus Creator/1  "1_J"
  Rate Transition13/1 -> Bus Creator/5  "polepair"
  Bus Creator/1 -> Out1/1
  Constant8/1 -> Data Type Conversion10/1
  Data Type Conversion9/1 -> Rate Transition12/1
  Rate Transition15/1 -> Bus Creator/2  "mu"
  J/1 -> Data Type Conversion12/1
  Data Type Conversion10/1 -> Rate Transition13/1
  mu/1 -> Data Type Conversion13/1
  M_R0/1 -> Data Type Conversion14/1
  Data Type Conversion13/1 -> Rate Transition15/1
  Constant7/1 -> Data Type Conversion9/1

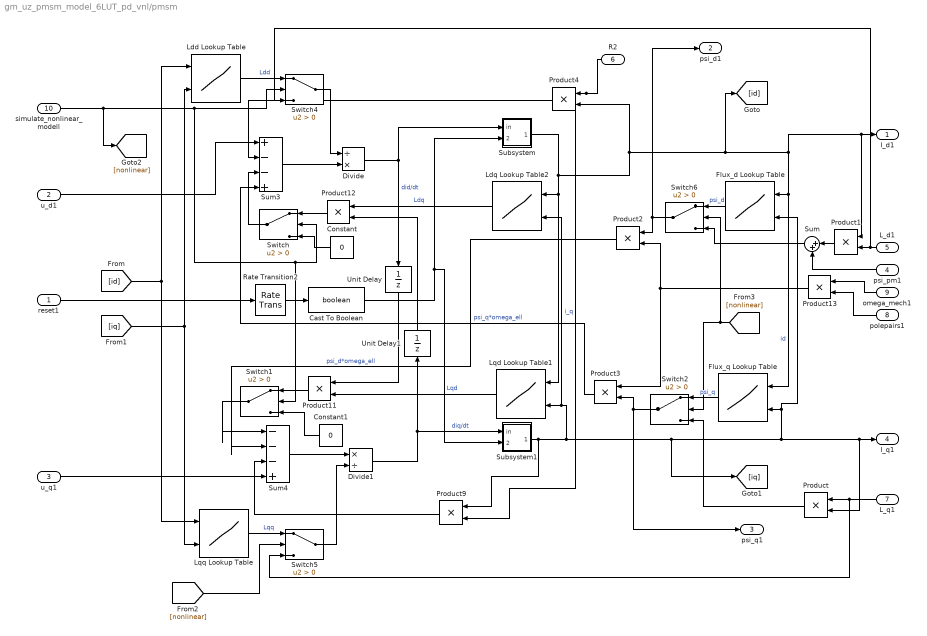
== system gm_uz_pmsm_model_6LUT_pd_vnl/pmsm ==
  reset1 : Inport
  u_d1 : Inport  Port=2
  u_q1 : Inport  Port=3
  psi_pm1 : Inport  Port=4
  L_d1 : Inport  Port=5
  R2 : Inport  Port=6
  L_q1 : Inport  Port=7
  polepairs1 : Inport  Port=8
  omega_mech1 : Inport  Port=9
  simulate_nonlinear_modell : Inport  Port=10
  Cast To Boolean : DataTypeConversion  OutDataTypeStr=boolean  SaturateOnIntegerOverflow=off  RndMeth=Floor
  Constant : Constant  Value=0  SampleTime=ts
  Constant1 : Constant  Value=0  SampleTime=ts
  Divide : Product  Inputs=/*
  Divide1 : Product  Inputs=*/
  Flux_d Lookup Table : Lookup_n-D  BreakpointsForDimension1=d_current_d_Flux  BreakpointsForDimension2=q_current_d_Flux  BreakpointsForDimension3=[5, 7]  Table=Flux_d  InternalRulePriority=Speed  RndMeth=Simplest
      settings: InputPortMap=u0,u1
  Flux_q Lookup Table : Lookup_n-D  BreakpointsForDimension1=d_current_q_Flux  BreakpointsForDimension2=q_current_q_Flux  BreakpointsForDimension3=[5, 7]  Table=Flux_q  InternalRulePriority=Speed  RndMeth=Simplest
      settings: InputPortMap=u0,u1
  Ldd Lookup Table : Lookup_n-D  BreakpointsForDimension1=d_current_q_Flux  BreakpointsForDimension2=q_current_q_Flux  BreakpointsForDimension3=[5, 7]  Table=Ldd  InternalRulePriority=Speed  RndMeth=Simplest
      settings: InputPortMap=u0,u1
  Ldq Lookup Table2 : Lookup_n-D  BreakpointsForDimension1=d_current_q_Flux  BreakpointsForDimension2=q_current_q_Flux  BreakpointsForDimension3=[5, 7]  Table=Ldq  InternalRulePriority=Speed  RndMeth=Simplest
      settings: InputPortMap=u0,u1
  Lqd Lookup Table1 : Lookup_n-D  BreakpointsForDimension1=d_current_q_Flux  BreakpointsForDimension2=q_current_q_Flux  BreakpointsForDimension3=[5, 7]  Table=Lqd  InternalRulePriority=Speed  RndMeth=Simplest
      settings: InputPortMap=u0,u1
  Lqq Lookup Table : Lookup_n-D  BreakpointsForDimension1=d_current_q_Flux  BreakpointsForDimension2=q_current_q_Flux  BreakpointsForDimension3=[5, 7]  Table=Lqq  InternalRulePriority=Speed  RndMeth=Simplest
      settings: InputPortMap=u0,u1
  Product{,1..4,9,11..13} (9 alike) : Product
  Rate Transition2 : RateTransition  OutPortSampleTime=ts
  Subsystem : Subsystem
  Subsystem1 : Subsystem
  Sum : Sum  Inputs=|++
  Sum3 : Sum  Inputs=|+--+
  Sum4 : Sum  Inputs=|---+
  Switch{,1..2,4..6} (6 alike) : Switch  Criteria=u2 > Threshold  SaturateOnIntegerOverflow=off  InputSameDT=off
  Unit Delay : UnitDelay  SampleTime=-1  HasFrameUpgradeWarning=on
  Unit Delay1 : UnitDelay  SampleTime=-1  HasFrameUpgradeWarning=on
  I_d1 : Outport
  psi_d1 : Outport  Port=2
  psi_q1 : Outport  Port=3
  I_q1 : Outport  Port=4
  wires:
  Sum4/1 -> Divide1/1
  u_q1/1 -> Sum4/4
  omega_mech1/1 -> Product13/1
  L_d1/1 -> Switch4/3, Product1/2
  Divide1/1 -> Unit Delay1/1, Subsystem1/1(in)  "diq/dt"
  polepairs1/1 -> Product13/2
  Product13/1 -> Product3/1, Product2/2
  Divide/1 -> Unit Delay/1, Subsystem/1(in)  "did/dt"
  Sum3/1 -> Divide/2
  Product9/1 -> Sum4/3
  Cast To Boolean/1 -> Subsystem/2(reset), Subsystem1/2(reset)
  u_d1/1 -> Sum3/1
  reset1/1 -> Rate Transition2/1
  Rate Transition2/1 -> Cast To Boolean/1
  R2/1 -> Product9/2, Product4/1
  Subsystem/1(outt) -> Lqd Lookup Table1/1, Ldq Lookup Table2/1, Product4/2, Flux_d Lookup Table/1, Flux_q Lookup Table/1, Product1/1, I_d1/1, [id]  "id"
  [id] -> Lqq Lookup Table/1, Ldd Lookup Table/1
  psi_pm1/1 -> Sum/2
  Subsystem1/1(outt) -> [iq], I_q1/1, Product/2, Flux_q Lookup Table/2, Flux_d Lookup Table/2, Ldq Lookup Table2/2, Lqd Lookup Table1/2, Product9/1  "i_q"
  [iq] -> Ldd Lookup Table/2, Lqq Lookup Table/2
  Product3/1 -> Sum3/4  "psi_q*omega_ell"
  Product4/1 -> Sum3/2
  Product2/1 -> Sum4/2  "psi_d*omega_ell"
  Unit Delay/1 -> Product11/1
  Unit Delay1/1 -> Product12/2
  Lqd Lookup Table1/1 -> Product11/2  "Lqd"
  Ldq Lookup Table2/1 -> Product12/1  "Ldq"
  Product12/1 -> Switch/1
  Switch/1 -> Sum3/3
  Constant/1 -> Switch/3
  Product11/1 -> Switch1/1
  Switch1/1 -> Sum4/1
  Constant1/1 -> Switch1/3
  L_q1/1 -> Switch5/3, Product/1
  Flux_q Lookup Table/1 -> Switch2/1  "psi_q"
  Switch2/1 -> psi_q1/1, Product3/2
  Product/1 -> Switch2/3
  Ldd Lookup Table/1 -> Switch4/1  "Ldd"
  Switch4/1 -> Divide/1
  Lqq Lookup Table/1 -> Switch5/1  "Lqq"
  Switch5/1 -> Divide1/2
  Flux_d Lookup Table/1 -> Switch6/1  "psi_d"
  Switch6/1 -> psi_d1/1, Product2/1
  Product1/1 -> Sum/1
  Sum/1 -> Switch6/3
  simulate_nonlinear_modell/1 -> [nonlinear], Switch/2, Switch1/2, Switch4/2
  [nonlinear] -> Switch5/2
  [nonlinear] -> Switch2/2, Switch6/2

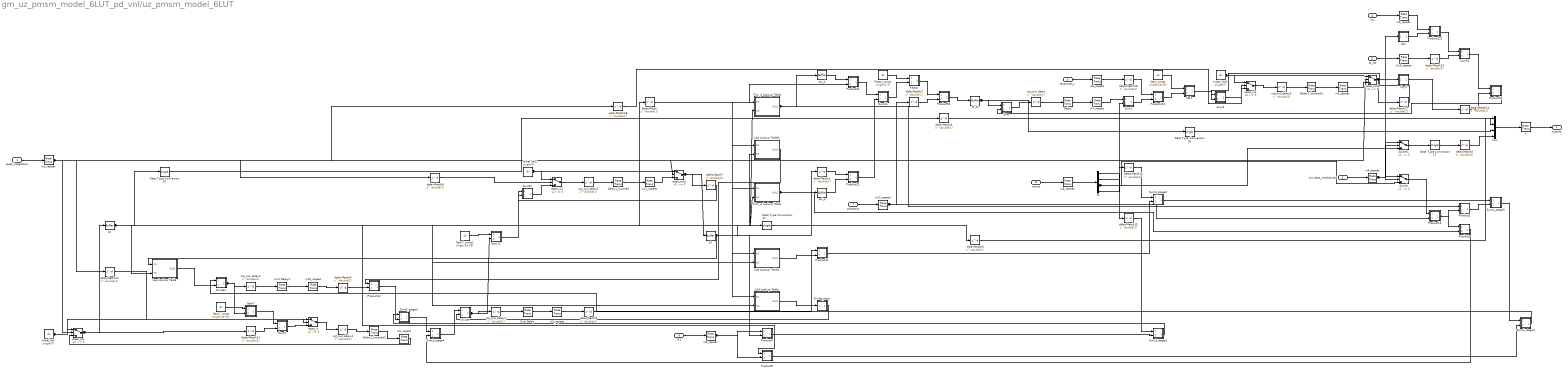
== system gm_uz_pmsm_model_6LUT_pd_vnl/uz_pmsm_model_6LUT ==
  reset_integrators : Inport  OutDataTypeStr=boolean  PortDimensions=1  SampleTime=2e-06
  simulate_mechanical : Inport  Port=2  OutDataTypeStr=boolean  PortDimensions=1  SampleTime=2e-06
  reciprocal_J : Inport  Port=3  OutDataTypeStr=single  PortDimensions=1  SampleTime=2e-06
  mu : Inport  Port=4  OutDataTypeStr=single  PortDimensions=1  SampleTime=2e-06
  M_n0 : Inport  Port=5  OutDataTypeStr=single  PortDimensions=1  SampleTime=2e-06
  R1 : Inport  Port=6  OutDataTypeStr=single  PortDimensions=1  SampleTime=2e-06
  polepairs : Inport  Port=7  OutDataTypeStr=single  PortDimensions=1  SampleTime=2e-06
  inputs : Inport  Port=8  OutDataTypeStr=single  PortDimensions=[4]  SampleTime=2e-06
  Abs : Subsystem
      mask Display: disp('NFP\nabs');
  Data Type Conversion{11,15..17} (4 alike) : DataTypeConversion  OutDataTypeStr=single
  Delay : RateTransition  OutPortSampleTimeOpt=Multiple of input port sample time  OutPortSampleTimeMultiple=200
  Delay1_lowered : RateTransition  OutPortSampleTimeOpt=Multiple of input port sample time  OutPortSampleTimeMultiple=200
  Delay1_lowered1 : RateTransition  OutPortSampleTimeOpt=Multiple of input port sample time  OutPortSampleTimeMultiple=200
  Delay1_lowered2 : RateTransition  OutPortSampleTimeOpt=Multiple of input port sample time  OutPortSampleTimeMultiple=200
  Divide : Subsystem
      mask Display: disp('NFP\nmul');
  Divide1 : Subsystem
      mask Display: disp('NFP\nmul');
  Divide_recip : Subsystem
      mask Display: disp('NFP\nmath');
  Factor : Subsystem
      mask Display: disp('NFP\nmul');
  Factor_const : Constant  Value=single(1.5)  OutDataTypeStr=single  SampleTime=1e-08
  Flux_d Lookup Table : Subsystem
  Flux_q Lookup Table : Subsystem
  Gain : Subsystem
      mask Display: disp('NFP\nmul');
  Gain7 : Subsystem
      mask Display: disp('NFP\nmul');
  Gain71 : Subsystem
      mask Display: disp('NFP\nmul');
  Gain7_const : Constant  Value=single(2e-06)  OutDataTypeStr=single  SampleTime=1e-08
  Gain7_const1 : Constant  Value=single(2e-06)  OutDataTypeStr=single  SampleTime=1e-08
  Gain_const : Constant  Value=single(2e-06)  OutDataTypeStr=single  SampleTime=1e-08
  Initial_Val : Constant  Value=single(0)  OutDataTypeStr=single  SampleTime=1e-08
  Initial_Val1 : Constant  Value=single(0)  OutDataTypeStr=single  SampleTime=1e-08
  Initial_Val2 : Constant  Value=single(0)  OutDataTypeStr=single  SampleTime=1e-08
  Ldd Lookup Table : Subsystem
  Ldq Lookup Table2 : Subsystem
  Lqd Lookup Table1 : Subsystem
  Lqq Lookup Table : Subsystem
  M_Mi : hdlmdlgenlib/Buffer
  Product11 : Subsystem
      mask Display: disp('NFP\nmul');
  Product111 : Subsystem
      mask Display: disp('NFP\nmul');
  Product12 : Subsystem
      mask Display: disp('NFP\nmul');
  Product121 : Subsystem
      mask Display: disp('NFP\nmul');
  Product13 : Subsystem
      mask Display: disp('NFP\nmul');
  Product2 : Subsystem
      mask Display: disp('NFP\nmul');
  Product21 : Subsystem
      mask Display: disp('NFP\nmul');
  Product3 : Subsystem
      mask Display: disp('NFP\nmul');
  Product31 : Subsystem
      mask Display: disp('NFP\nmul');
  Product4 : Subsystem
      mask Display: disp('NFP\nmul');
  Product41 : Subsystem
      mask Display: disp('NFP\nmul');
  Product9 : Subsystem
      mask Display: disp('NFP\nmul');
  Product91 : Subsystem
      mask Display: disp('NFP\nmul');
  Sign1 : Subsystem
      mask Display: disp('NFP\nsignum');
  Sum : Subsystem
      mask Display: disp('NFP\nadd');
  Sum1 : Subsystem
      mask Display: disp('NFP\nadd');
  Sum3 : Subsystem
      mask Display: disp('NFP\nadd');
  Sum31 : Subsystem
      mask Display: disp('NFP\nadd');
  Sum3_stage2 : Subsystem
      mask Display: disp('NFP\nadd');
  Sum3_stage3 : Subsystem
      mask Display: disp('NFP\nadd');
  Sum3_stage4 : Subsystem
      mask Display: disp('NFP\nadd');
  Sum4_stage2 : Subsystem
      mask Display: disp('NFP\nadd');
  Sum4_stage3 : Subsystem
      mask Display: disp('NFP\nadd');
  Sum4_stage4 : Subsystem
      mask Display: disp('NFP\nadd');
  Sum5 : Subsystem
      mask Display: disp('NFP\nadd');
  Sum51 : Subsystem
      mask Display: disp('NFP\nadd');
  Sum52 : Subsystem
      mask Display: disp('NFP\nadd');
  Switch : Switch  Criteria=u2 ~= 0  Threshold=double(0)  OutDataTypeStr=single  SampleTime=1e-08  SaturateOnIntegerOverflow=off  InputSameDT=off
  Switch1 : Switch  Criteria=u2 ~= 0  Threshold=double(0)  OutDataTypeStr=single  SampleTime=1e-08  SaturateOnIntegerOverflow=off  InputSameDT=off
  Unit Delay : RateTransition  OutPortSampleTimeOpt=Multiple of input port sample time  OutPortSampleTimeMultiple=200
  Unit Delay1 : RateTransition  OutPortSampleTimeOpt=Multiple of input port sample time  OutPortSampleTimeMultiple=200
  crp_out_delay{,1..5} (6 alike) : Delay  DelayLength=double(1)  InitialCondition=0  SampleTime=1e-08
  delayMatch{,1..18} (19 alike) : Delay  DelayLength=double(1)  InitialCondition=0  SampleTime=1e-08
  in0_repeat : RateTransition  Integrity=off  Deterministic=off  OutPortSampleTimeOpt=Multiple of input port sample time  OutPortSampleTimeMultiple=1/200
  in10_repeat : RateTransition  Integrity=off  Deterministic=off  OutPortSampleTimeOpt=Multiple of input port sample time  OutPortSampleTimeMultiple=1/200
  in11_repeat : RateTransition  Integrity=off  Deterministic=off  OutPortSampleTimeOpt=Multiple of input port sample time  OutPortSampleTimeMultiple=1/200
  in12_repeat : RateTransition  Integrity=off  Deterministic=off  OutPortSampleTimeOpt=Multiple of input port sample time  OutPortSampleTimeMultiple=1/200
  in13_repeat : RateTransition  Integrity=off  Deterministic=off  OutPortSampleTimeOpt=Multiple of input port sample time  OutPortSampleTimeMultiple=1/200
  in1_repeat : RateTransition  Integrity=off  Deterministic=off  OutPortSampleTimeOpt=Multiple of input port sample time  OutPortSampleTimeMultiple=1/200
  in2_repeat : RateTransition  Integrity=off  Deterministic=off  OutPortSampleTimeOpt=Multiple of input port sample time  OutPortSampleTimeMultiple=1/200
  in3_repeat : RateTransition  Integrity=off  Deterministic=off  OutPortSampleTimeOpt=Multiple of input port sample time  OutPortSampleTimeMultiple=1/200
  in4_repeat : RateTransition  Integrity=off  Deterministic=off  OutPortSampleTimeOpt=Multiple of input port sample time  OutPortSampleTimeMultiple=1/200
  in5_repeat : RateTransition  Integrity=off  Deterministic=off  OutPortSampleTimeOpt=Multiple of input port sample time  OutPortSampleTimeMultiple=1/200
  in6_repeat : RateTransition  Integrity=off  Deterministic=off  OutPortSampleTimeOpt=Multiple of input port sample time  OutPortSampleTimeMultiple=1/200
  in7_repeat : RateTransition  Integrity=off  Deterministic=off  OutPortSampleTimeOpt=Multiple of input port sample time  OutPortSampleTimeMultiple=1/200
  in8_repeat : RateTransition  Integrity=off  Deterministic=off  OutPortSampleTimeOpt=Multiple of input port sample time  OutPortSampleTimeMultiple=1/200
  in9_repeat : RateTransition  Integrity=off  Deterministic=off  OutPortSampleTimeOpt=Multiple of input port sample time  OutPortSampleTimeMultiple=1/200
  mux : Mux
  psi_d : hdlmdlgenlib/Buffer
  psi_q : hdlmdlgenlib/Buffer
  reset_in : Switch  Criteria=u2 ~= 0  Threshold=double(0)  OutDataTypeStr=single  SampleTime=1e-08  SaturateOnIntegerOverflow=off  InputSameDT=off
  reset_in1 : Switch  Criteria=u2 ~= 0  Threshold=double(0)  OutDataTypeStr=single  SampleTime=1e-08  SaturateOnIntegerOverflow=off  InputSameDT=off
  reset_in2 : Switch  Criteria=u2 ~= 0  Threshold=double(0)  OutDataTypeStr=single  SampleTime=1e-08  SaturateOnIntegerOverflow=off  InputSameDT=off
  reset_out : Switch  Criteria=u2 ~= 0  Threshold=double(0)  OutDataTypeStr=single  SampleTime=1e-08  SaturateOnIntegerOverflow=off  InputSameDT=off
  reset_out1 : Switch  Criteria=u2 ~= 0  Threshold=double(0)  OutDataTypeStr=single  SampleTime=1e-08  SaturateOnIntegerOverflow=off  InputSameDT=off
  reset_out2 : Switch  Criteria=u2 ~= 0  Threshold=double(0)  OutDataTypeStr=single  SampleTime=1e-08  SaturateOnIntegerOverflow=off  InputSameDT=off
  t : RateTransition  OutPortSampleTimeOpt=Multiple of input port sample time  OutPortSampleTimeMultiple=200
  t1 : Demux
  t2 : hdlmdlgenlib/Buffer
  t3 : hdlmdlgenlib/Buffer
  outputs : Outport  SampleTime=2e-06
  wires:
  reset_out1/1 -> Switch1/1, Switch/1, Sign1/1(In1), Abs/1(In1), delayMatch17/1
  delayMatch12/1 -> reset_in/2
  delayMatch11/1 -> Sum5/2(In2)
  delayMatch8/1 -> reset_in2/2
  delayMatch7/1 -> Sum51/2(In2)
  delayMatch3/1 -> mux/1
  delayMatch2/1 -> Product91/2(In2)
  Gain/1(Out1) -> Sum3/1(In1)
  Product31/1(Out1) -> Sum31/1(In1)
  Sum31/1(Out1) -> Factor/2(In2)
  Sum/1(Out1) -> crp_out_delay/1
  Product41/1(Out1) -> Sum/2(In2)
  Sum52/1(Out1) -> Product41/1(In1)
  Product121/1(Out1) -> Sum52/1(In1)
  Abs/1(Out1) -> Product121/2(In2)
  Sign1/1(Out1) -> delayMatch14/1
  Product13/1(Out1) -> Product2/2(In2), Product3/1(In1)
  Sum3_stage4/1(Out1) -> Divide/1(In1)
  Sum3_stage3/1(Out1) -> Sum3_stage4/1(In1)
  Sum3_stage2/1(Out1) -> Sum3_stage3/1(In1)
  Divide_recip/1(Out1) -> Divide/2(In2)
  Sum51/1(Out1) -> reset_in2/3
  Product4/1(Out1) -> Sum3_stage2/2(In2)
  Product21/1(Out1) -> Sum31/2(In2)
  Product12/1(Out1) -> Sum3_stage3/2(In2)
  Product9/1(Out1) -> Sum4_stage4/2(In2)
  Sum4_stage4/1(Out1) -> Divide1/1(In1)
  Sum4_stage3/1(Out1) -> Sum4_stage4/1(In1)
  Sum4_stage2/1(Out1) -> Sum4_stage3/1(In1)
  Sum1/1(Out1) -> Product111/2(In2)
  Product111/1(Out1) -> Gain/2(In2)
  Sum3/1(Out1) -> reset_in1/3
  Product11/1(Out1) -> Sum4_stage2/2(In2)
  Sum5/1(Out1) -> reset_in/3
  reset_out/1 -> delayMatch11/1, t2/1
  reset_out2/1 -> delayMatch7/1, t3/1
  Data Type Conversion17/1 -> delayMatch5/1
  Data Type Conversion15/1 -> delayMatch4/1
  Data Type Conversion11/1 -> delayMatch3/1
  delayMatch13/1 -> Sum52/2(In2)
  delayMatch16/1 -> Product111/1(In1)
  delayMatch18/1 -> reset_in1/2
  Factor_const/1 -> Factor/1(In1)
  Gain7_const1/1 -> Gain71/1(In1)
  Gain_const/1 -> Gain/1(In1)
  Gain7_const/1 -> Gain7/1(In1)
  t1/2 -> delayMatch10/1
  t1/1 -> delayMatch15/1
  delayMatch6/1 -> Product12/2(In2)
  delayMatch9/1 -> Product11/1(In1)
  delayMatch4/1 -> mux/2
  delayMatch/1 -> Product31/2(In2)
  Factor/1(Out1) -> Product91/1(In1)
  Product91/1(Out1) -> M_Mi/1
  M_Mi/1 -> Data Type Conversion16/1, Sum/1(In1)
  delayMatch14/1 -> Product41/2(In2)
  Switch/1 -> Product13/1(In1)
  Product3/1(Out1) -> Sum3_stage4/2(In2)
  Divide/1(Out1) -> crp_out_delay1/1, Gain71/2(In2)
  Gain71/1(Out1) -> Sum51/1(In1)
  reset_in2/1 -> crp_out_delay2/1
  Initial_Val2/1 -> reset_in2/1, reset_out2/1
  t3/1 -> Data Type Conversion11/1, delayMatch1/1, Lqq Lookup Table/1(In1), Lqd Lookup Table1/1(In1), Ldq Lookup Table2/1(In1), Ldd Lookup Table/1(In1), Flux_q Lookup Table/1(In1), Flux_d Lookup Table/1(In1), Product4/2(In2)
  delayMatch1/1 -> Product21/1(In1)
  psi_q/1 -> Product21/2(In2)
  Flux_q Lookup Table/1(Out1) -> psi_q/1, Product3/2(In2)
  t2/1 -> Data Type Conversion15/1, delayMatch/1, Lqq Lookup Table/2(In2), Lqd Lookup Table1/2(In2), Ldq Lookup Table2/2(In2), Ldd Lookup Table/2(In2), Flux_q Lookup Table/2(In2), Flux_d Lookup Table/2(In2), Product9/1(In1)
  Ldq Lookup Table2/1(Out1) -> Product12/1(In1)
  Ldd Lookup Table/1(Out1) -> Divide_recip/1(In1)
  t1/4 -> Sum1/2(In2)
  t1/3 -> Switch1/3, Switch/3
  delayMatch10/1 -> Sum4_stage2/1(In1)
  delayMatch15/1 -> Sum3_stage2/1(In1)
  reset_in1/1 -> crp_out_delay5/1
  Initial_Val1/1 -> reset_in1/1, reset_out1/1
  delayMatch17/1 -> Sum3/2(In2)
  Switch1/1 -> Data Type Conversion17/1
  delayMatch5/1 -> mux/4
  Product2/1(Out1) -> Sum4_stage3/2(In2)
  Flux_d Lookup Table/1(Out1) -> psi_d/1, Product2/1(In1)
  psi_d/1 -> Product31/1(In1)
  Lqd Lookup Table1/1(Out1) -> Product11/2(In2)
  Divide1/1(Out1) -> crp_out_delay3/1, Gain7/2(In2)
  Lqq Lookup Table/1(Out1) -> Divide1/2(In2)
  Gain7/1(Out1) -> Sum5/1(In1)
  reset_in/1 -> crp_out_delay4/1
  Initial_Val/1 -> reset_in/1, reset_out/1
  Data Type Conversion16/1 -> mux/3
  crp_out_delay5/1 -> Delay1_lowered1/1
  crp_out_delay4/1 -> Delay1_lowered2/1
  crp_out_delay3/1 -> Unit Delay1/1
  crp_out_delay2/1 -> Delay1_lowered/1
  crp_out_delay1/1 -> Unit Delay/1
  crp_out_delay/1 -> Delay/1
  in2_repeat/1 -> reset_out/3
  Delay1_lowered2/1 -> in2_repeat/1
  in3_repeat/1 -> delayMatch9/1
  Unit Delay/1 -> in3_repeat/1
  in5_repeat/1 -> reset_out1/3
  Delay1_lowered1/1 -> in5_repeat/1
  in7_repeat/1 -> Sum1/1(In1)
  Delay/1 -> in7_repeat/1
  in10_repeat/1 -> delayMatch6/1
  Unit Delay1/1 -> in10_repeat/1
  in11_repeat/1 -> reset_out2/3
  Delay1_lowered/1 -> in11_repeat/1
  mux/1 -> t/1
  in13_repeat/1 -> delayMatch13/1
  in12_repeat/1 -> delayMatch2/1, Product13/2(In2)
  in9_repeat/1 -> Product9/2(In2), Product4/1(In1)
  in8_repeat/1 -> t1/1
  in6_repeat/1 -> delayMatch16/1
  in4_repeat/1 -> Switch1/2, Switch/2
  in1_repeat/1 -> reset_out/2, reset_out2/2, reset_out1/2, delayMatch8/1, delayMatch12/1, delayMatch18/1
  in0_repeat/1 -> Product121/1(In1)
  t/1 -> outputs/1
  inputs/1 -> in8_repeat/1
  polepairs/1 -> in12_repeat/1
  R1/1 -> in9_repeat/1
  M_n0/1 -> in13_repeat/1
  mu/1 -> in0_repeat/1
  reciprocal_J/1 -> in6_repeat/1
  simulate_mechanical/1 -> in4_repeat/1
  reset_integrators/1 -> in1_repeat/1
